simulink model "ABS"  (R2018a)
settings: Solver=VariableStepAuto  StartTime=0.0  StopTime=10.0  RelTol=1e-3
undefined symbols (not defined in the file): g, I, m, R, v0
settings Model: Creator=NZT48  LastModifiedBy=NZT48

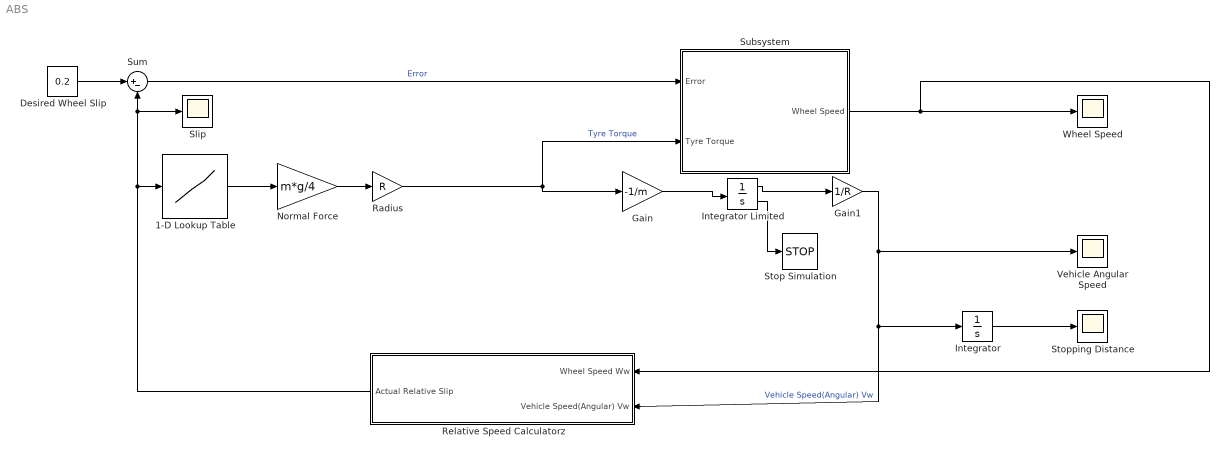
== system ABS ==
  1-D Lookup Table : Lookup_n-D  NumberOfTableDimensions=1  BreakpointsForDimension1=[0,0.05,0.1,0.15,0.21,0.25,0.3,0.35,0.4,0.45,0.5,0.55,0.6,0.65,0.7,0.75,0.8,0.85,0.9,0.95,1]  Table=[0,0.4,0.8,0.97,1,0.98,0.96,0.94,0.92,0.9,0.88,0.855,0.83,0.81,0.79,0.77,0.75,0.71,0.72,0.71,0.7]  InternalRulePriority=Speed  RndMeth=Simplest  InputSameDT=on
  Desired Wheel Slip : Constant  Value=0.2
  Gain : Gain  Gain=-1/m
  Gain1 : Gain  Gain=1/R
  Integrator : Integrator
  Integrator Limited : Integrator  InitialCondition=v0  LimitOutput=on  UpperSaturationLimit=1000  LowerSaturationLimit=0  ShowSaturationPort=on
  "Normal Force " : Gain  Gain=m*g/4
  Radius : Gain  Gain=R
  Relative Speed Calculatorz : Subsystem
  Slip : Scope
  Stop Simulation : Stop
  Stopping Distance : Scope
  Subsystem : Subsystem
  Sum : Sum  Inputs=|+-
  "Vehicle Angular Speed " : Scope
  Wheel Speed : Scope
  wires:
  Desired Wheel Slip/1 -> Sum/1
  1-D Lookup Table/1 -> "Normal Force "/1
  "Normal Force "/1 -> Radius/1
  Sum/1 -> Subsystem/1(Error)  "Error"
  Radius/1 -> Gain/1, Subsystem/2(Tyre Torque)  "Tyre Torque"
  Subsystem/1(Wheel Speed) -> Wheel Speed/1, Relative Speed Calculatorz/1(Wheel Speed Ww)
  Gain/1 -> Integrator Limited/1
  Integrator Limited/1 -> Gain1/1
  Gain1/1 -> Relative Speed Calculatorz/2(Vehicle Speed(Angular) Vw), Integrator/1, "Vehicle Angular Speed "/1  "Vehicle Speed(Angular) Vw"
  Integrator Limited/2 -> Stop Simulation/1
  Integrator/1 -> Stopping Distance/1
  Relative Speed Calculatorz/1("Actual Relative Slip ") -> 1-D Lookup Table/1, Slip/1, Sum/2

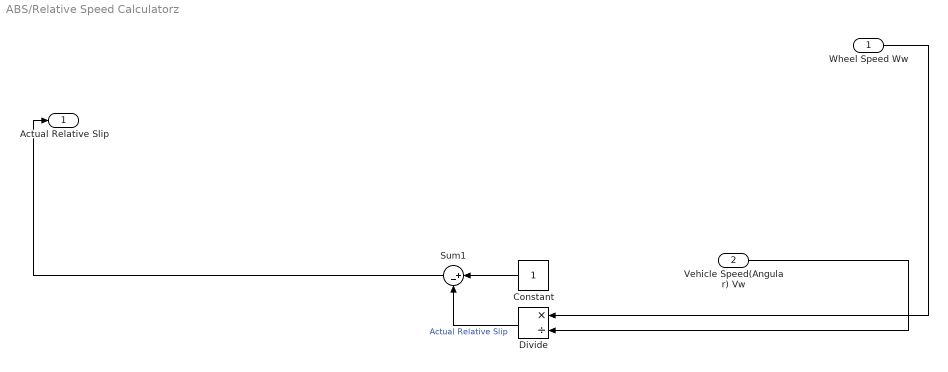
== system ABS/Relative Speed Calculatorz ==
  Wheel Speed Ww : Inport
  Vehicle Speed(Angular) Vw : Inport  Port=2
  Constant : Constant
  Divide : Product  Inputs=*/
  Sum1 : Sum  Inputs=|+-
  "Actual Relative Slip " : Outport
  wires:
  Constant/1 -> Sum1/1
  Divide/1 -> Sum1/2  "Actual Relative Slip"
  Wheel Speed Ww/1 -> Divide/1
  Sum1/1 -> "Actual Relative Slip "/1
  Vehicle Speed(Angular) Vw/1 -> Divide/2

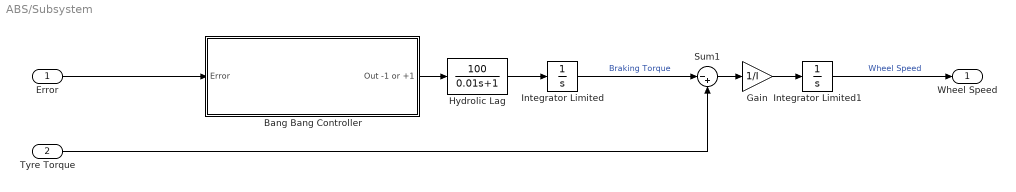
== system ABS/Subsystem ==
  Error : Inport
  Tyre Torque : Inport  Port=2
  "Bang Bang Controller " : Subsystem
  Gain : Gain  Gain=1/I
  "Hydrolic Lag " : TransferFcn  Numerator=[100]  Denominator=[0.01 1]
  Integrator Limited : Integrator  LimitOutput=on  UpperSaturationLimit=1000  LowerSaturationLimit=0
  Integrator Limited1 : Integrator  InitialCondition=v0/R  LimitOutput=on  UpperSaturationLimit=1000  LowerSaturationLimit=0
  Sum1 : Sum  Inputs=|-+
  Wheel Speed : Outport
  wires:
  Integrator Limited/1 -> Sum1/1  "Braking Torque"
  Sum1/1 -> Gain/1
  Tyre Torque/1 -> Sum1/2
  Gain/1 -> Integrator Limited1/1
  "Hydrolic Lag "/1 -> Integrator Limited/1
  Error/1 -> "Bang Bang Controller "/1(Error)
  Integrator Limited1/1 -> Wheel Speed/1  "Wheel Speed"
  "Bang Bang Controller "/1(Out -1 or +1) -> "Hydrolic Lag "/1

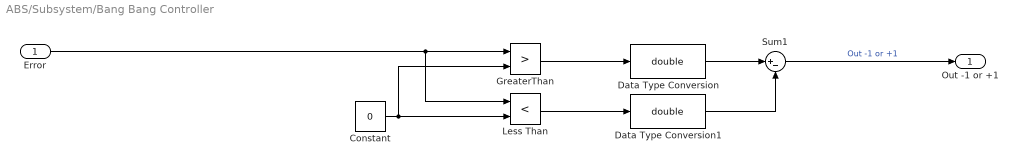
== system ABS/Subsystem/Bang Bang Controller  ==
  Error : Inport
  Constant : Constant  Value=0
  Data Type Conversion : DataTypeConversion  OutDataTypeStr=double  RndMeth=Zero
  Data Type Conversion1 : DataTypeConversion  OutDataTypeStr=double  RndMeth=Zero
  GreaterThan : RelationalOperator  Operator=>  OutDataTypeStr=boolean  RndMeth=Simplest
  Less Than : RelationalOperator  Operator=<  OutDataTypeStr=boolean  RndMeth=Simplest
  Sum1 : Sum  Inputs=|+-
  Out -1 or +1 : Outport
  wires:
  Data Type Conversion/1 -> Sum1/1
  GreaterThan/1 -> Data Type Conversion/1
  Error/1 -> Less Than/1, GreaterThan/1
  Data Type Conversion1/1 -> Sum1/2
  Less Than/1 -> Data Type Conversion1/1
  Constant/1 -> GreaterThan/2, Less Than/2
  Sum1/1 -> Out -1 or +1/1  "Out -1 or +1"
